simulink model "usv_6dof"  (R2023b)
settings: Solver=VariableStepAuto  StartTime=0.0  StopTime=200  RelTol=1e-3
libraries: slpidlib x1
settings Model: Creator=hw  LastModifiedBy=hw

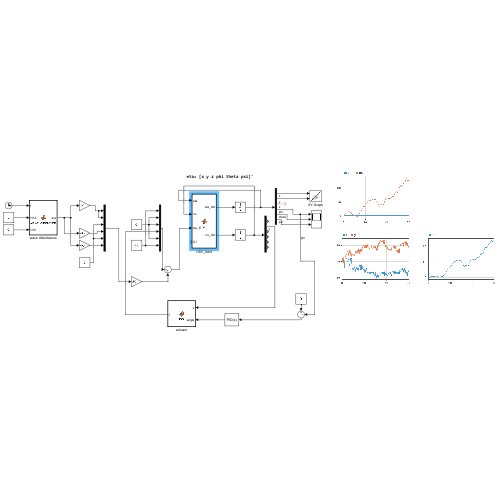
[thumbnail: Simulink's stored preview of the top-level diagram]
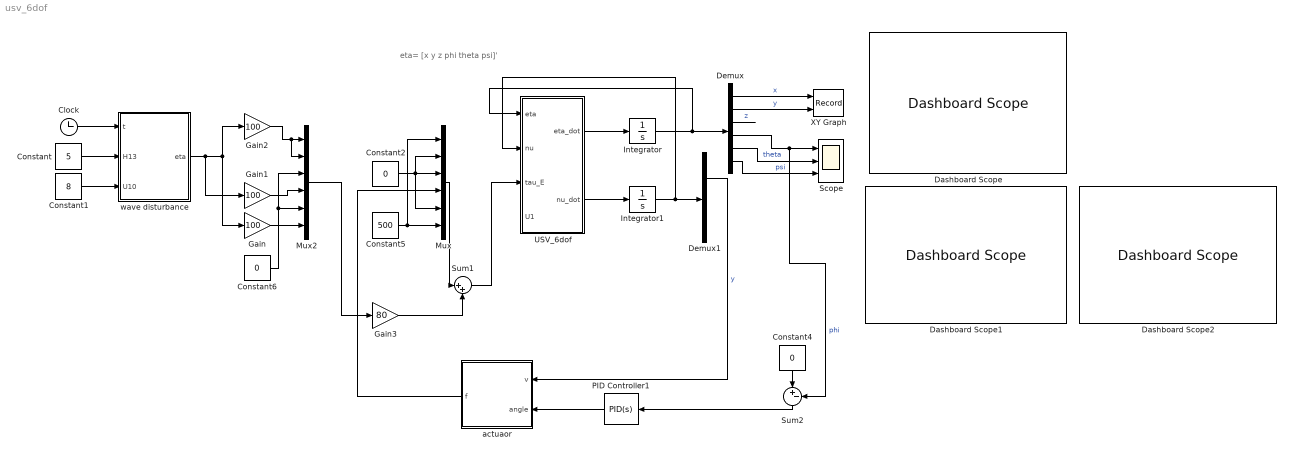
== system usv_6dof ==
  note: eta= [x y z phi theta psi]'
  Clock : Clock
  Constant : Constant  Value=5
  Constant1 : Constant  Value=8
  Constant2 : Constant  Value=0
  Constant4 : Constant  Value=0
  Constant5 : Constant  Value=500
  Constant6 : Constant  Value=0
  Dashboard Scope : DashboardScope
  Dashboard Scope1 : DashboardScope
  Dashboard Scope2 : DashboardScope
  Demux : Demux  Outputs=6
  Demux1 : Demux  Outputs=6
  Gain : Gain  Gain=100
  Gain1 : Gain  Gain=100
  Gain2 : Gain  Gain=100
  Gain3 : Gain  Gain=80
  Integrator : Integrator
  Integrator1 : Integrator
  Mux : Mux  Inputs=6
  Mux2 : Mux  Inputs=6
  PID Controller1 : slpidlib/PID Controller  Controller=PID  Form=Parallel  TimeDomain=Continuous-time  UseExternalTs=off  SampleTime=-1  IntegratorMethod=Forward Euler  FilterMethod=Forward Euler  ControllerParametersSource=internal  P=5  I=3  UseKiTs=off  D=2  N=100  UseFilter=on  TunerSelectOption=Transfer Function Based (PID Tuner App)  InitialConditionSource=internal  InitialConditionForIntegrator=0  InitialConditionForFilter=0  DifferentiatorICPrevScaledInput=0  ExternalReset=none  TrackingMode=off  Kt=1  LimitOutput=off  SatLimitsSource=internal  UpperSaturationLimit=inf  LowerSaturationLimit=-inf  LinearizeAsGain=on  AntiWindupMode=none  Kb=1  LimitIntegrator=off  UpperIntegratorSaturationLimit=inf  LowerIntegratorSaturationLimit=-inf  POutMin=[]  POutMax=[]  IOutMin=[]  IOutMax=[]  DOutMin=[]  DOutMax=[]  NOutMin=[]  NOutMax=[]  SumOutMin=[-15]  SumOutMax=[15]  SaturationOutMin=[]  SaturationOutMax=[]  PParamMin=[]  PParamMax=[]  IParamMin=[]  IParamMax=[]  DParamMin=[]  DParamMax=[]  NParamMin=[]  NParamMax=[]  KbParamMin=[]  KbParamMax=[]  KtParamMin=[]  KtParamMax=[]  KbOutMin=[]  KbOutMax=[]  KtOutMin=[]  KtOutMax=[]  IntegratorOutMin=[]  IntegratorOutMax=[]  FilterOutMin=[]  FilterOutMax=[]  SumI1OutMin=[]  SumI1OutMax=[]  SumI2OutMin=[]  SumI2OutMax=[]  SumI3OutMin=[]  SumI3OutMax=[]  SumI4OutMin=[]  SumI4OutMax=[]  SumDOutMin=[]  SumDOutMax=[]  DifferentiatorOutMin=[]  DifferentiatorOutMax=[]  FilterDiffOutCoefMin=[]  FilterDiffOutCoefMax=[]  ReciprocalOutMin=[]  ReciprocalOutMax=[]  SumDenOutMin=[]  SumDenOutMax=[]  SumNumOutMin=[]  SumNumOutMax=[]  DivideOutMin=[]  DivideOutMax=[]  UdiffTsProdOutMin=[]  UdiffTsProdOutMax=[]  NTsProdOutMin=[]  NTsProdOutMax=[]  UintegralTsProdOutMin=[]  UintegralTsProdOutMax=[]  UngainTsProdOutMin=[]  UngainTsProdOutMax=[]  ClampingZeroOutDataTypeStr=Inherit: Inherit via back propagation  ClampingZeroOutMin=[]  ClampingZeroOutMax=[]  FilterDenConstantOutDataTypeStr=Inherit: Inherit via back propagation  FilterDenConstantOutMin=[]  FilterDenConstantOutMax=[]  PCopyOutDataTypeStr=Inherit: Inherit via back propagation  PCopyOutMin=[]  PCopyOutMax=[]  NCopyOutDataTypeStr=Inherit: Inherit via back propagation  NCopyOutMin=[]  NCopyOutMax=[]  IntegratorContinuousStateAttributes=''  IntegratorStateMustResolveToSignalObject=off  IntegratorRTWStateStorageClass=Auto  FilterContinuousStateAttributes=''  FilterStateMustResolveToSignalObject=off  FilterRTWStateStorageClass=Auto  ParallelPVariant=InternalParameters  IdealPVariant=Disabled  IVariant=InternalParameters  DVariant=InternalParameters  IntegratorVariant=Continuous  SatVariant=Disabled  AWVariant=Passthrough  PCopyVariant=Disabled  TRVariant=Disabled  FdbkBlocksVariant=Forward  IdealPFdbkVariant=Disabled  SatFdbkVariant=Disabled  DerivativeFilterVariant=ContFilter  NVariant=InternalParameters  NCopyVariant=Disabled  FilterICVariant=InternalICsFilter  IntegratorICVariant=InternalICs  ExternalResetVariant=Disabled  TRSumVariant=Passthrough  SumFdbkVariant=Disabled  SumVariant=Sum_PID  TsampFilterVariant=InternalTs  TsampNgainVariant=Passthrough  TsampIntegralVariant=Disabled_SignalSpec  ExternalSaturationOutDataTypeStr=Inherit: Same as second input
  Scope : Scope  NumInputPorts=3
  Sum1 : Sum  Inputs=|++
  Sum2 : Sum  Inputs=|+-
  USV_6dof : MATLAB Function  TreatAsAtomicUnit=on
  XY Graph : Record  FileSettingsInternal="{\"entries\":[{\"content\":{\"excelSettings\":{\"content\":{},\"type\":\"Streamout.ExcelSettings\"}},\"type\":\"Streamout.FileSettingStorage\",\"uuid\":\"\"}],\"packageUris\":[\"http:\\/\\/schema.mathworks.com\\/mf0\\/streamout_blocks\\/R2020a\"],\"version\":\"1.0\"}"  Layout=[1 1]  SignalsInternal="{\"entries\":[{\"content\":{\"signals\":[{\"content\":{\"blockPath\":[],\"dimensions\":[1],\"domain\":\"\",\"lineColor\":\"#a2142f\",\"plots\":[1],\"port\":1,\"sid\":[\"\"],\"signalID\":11724,\"signalName\":\"x\"},\"type\":\"RecordBlkView.Signal\",\"uuid\":\"\"},{\"content\":{\"blockPath\":[],\"dimensions\":[1],\"domain\":\"\",\"lineColor\":\"#139fff\",\"plots\":[1],\"port\":2,\"sid\":[\"\"],\"signalID\":11728,\"signalName\":\"y\"},\"type\":\"RecordBlkView.Signal\",\"uuid\":\"\"}]},\"type\":\"RecordBlkView.InputSignals\",\"uuid\":\"\"}],\"packageUris\":[\"http:\\/\\/schema.mathworks.com\\/mf0\\/streamout_blocks\\/R2020a\"],\"version\":\"1.0\"}"  VisualizationBindings="{\"xyplotplugin\":{\"info\":[{\"series\":[{\"bindingParametersList\":[{\"parameter\":\"X-Axis\",\"signalID\":11724,\"signalName\":\"x\"},{\"parameter\":\"Y-Axis\",\"signalID\":11728,\"signalName\":\"y\"}],\"seriesID\":30360}],\"subplotID\":1}]}}"  CompatibilityTag=XY
  actuaor : MATLAB Function  TreatAsAtomicUnit=on
  wave disturbance : MATLAB Function  TreatAsAtomicUnit=on
  wires:
  wave disturbance/1(eta) -> Gain1/1, Gain2/1, Gain/1
  USV_6dof/2(nu_dot) -> Integrator1/1
  Constant/1 -> wave disturbance/2(H13)
  Integrator1/1 -> Demux1/1, USV_6dof/2(nu)
  Integrator/1 -> USV_6dof/1(eta), Demux/1
  Clock/1 -> wave disturbance/1(t)
  USV_6dof/1(eta_dot) -> Integrator/1
  Constant1/1 -> wave disturbance/3(U10)
  Demux/1 -> XY Graph/1  "x"
  Demux/2 -> XY Graph/2  "y"
  Demux/3 -> ?  "z"
  Demux/5 -> Scope/2  "theta"
  Demux/6 -> Scope/3  "psi"
  Constant2/1 -> Mux/5, Mux/2, Mux/3
  Constant5/1 -> Mux/6, Mux/1
  Mux/1 -> Sum1/1
  Gain2/1 -> Mux2/2, Mux2/1
  Gain/1 -> Mux2/6
  Mux2/1 -> Gain3/1
  Sum1/1 -> USV_6dof/3(tau_E)
  Gain1/1 -> Mux2/4
  Constant6/1 -> Mux2/5, Mux2/3
  Gain3/1 -> Sum1/2
  actuaor/1(f) -> Mux/4
  PID Controller1/1 -> actuaor/2(angle)
  Constant4/1 -> Sum2/1
  Demux/4 -> Sum2/2, Scope/1  "phi"
  Sum2/1 -> PID Controller1/1
  Demux1/2 -> actuaor/1(v)  "y"

== matlab function usv_6dof/actuaor ==
  data: v input; angle input size=1*1; f output size=1*1
function f  = top(v, angle)

f=1/2*v^2*1025*angle*10;
end

== matlab function usv_6dof/USV_6dof ==
  data: eta input size=6*1; eta_dot output size=6*1; nu input size=6*1; nu_dot output size=6*1; tau_E input size=6*1; U1 input
function [eta_dot,nu_dot]= fcn(eta,nu,tau_E,U1)
%%定义常量
    m=37;     %船体质量
    g = 9.81; % 重力加速度, m/s^2
    rho = 1025; % 海水密度, kg/m^3
    r_G=[0,0,0]'; %质心坐标
    r_f=[0 0 0]';  %浮心坐标
    I0=[0.11 0.11 0.11;0.22 0.22 0.22;0.33 0.33 0.33];  %转动惯量
    V=0.4562;  %排水体积
    W=m*g;
    B=W;
    % % B=rho*g*V;
%%定义位置与姿态等
    x=eta(1);
    y=eta(2);
    z=eta(3);
    phi=eta(4);
    theta=eta(5);
    psi=eta(6);

    u=nu(1);
    v=nu(2);
    w=nu(3);
    p=nu(4);
    q=nu(5);
    r=nu(6);
    
    x_g=r_G(1);
    y_g=r_G(2);
    z_g=r_G(3);

    x_f=r_f(1);
    y_f=r_f(2);
    z_f=r_f(3);

    % 转动惯量
    I_x = I0(1,1); % 绕x轴的转动惯量
    I_y = I0(2,2); % 绕y轴的转动惯量
    I_z = I0(3,3); % 绕z轴的转动惯量
    I_xy = -I0(1,2); % x-y平面的惯性积
    I_xz = -I0(1,3); % x-z平面的惯性积
    I_yz = -I0(2,3); % y-z平面的惯性积
%%定义转换矩阵
    J_eta = [cos(psi)*cos(theta), -sin(psi)*cos(phi) + cos(psi)*sin(theta)*sin(phi), sin(psi)*sin(phi) + cos(psi)*cos(phi)*sin(theta),0,0,0;
              sin(psi)*cos(theta), cos(psi)*cos(phi) + sin(psi)*sin(theta)*sin(phi), -cos(psi)*sin(phi) + sin(psi)*cos(phi)*sin(theta),0,0,0;
              -sin(theta), cos(theta)*sin(phi), cos(theta)*cos(phi),0,0,0;
              0,0,0,1,sin(phi)*tan(theta),cos(phi)*tan(theta);
              0,0,0,0,cos(phi),-sin(phi);
              0,0,0,0,sin(phi)/cos(theta),cos(phi)/cos(theta)]; 
  % 刚体质量矩阵
    M_RB = [
        m,   0,   0,   0,  m*z_g, -m*y_g;
        0,   m,   0,  -m*z_g, 0,  m*x_g;
        0,   0,   m,  m*y_g, -m*x_g, 0;
        0,  -m*z_g, m*y_g, I_x, -I_xy, -I_xz;
        m*z_g, 0,  -m*x_g, -I_xy, I_y, -I_yz;
        -m*y_g, m*x_g, 0, -I_xz, -I_yz, I_z];
  
   
        A11 =1000;  % 附加质量，沿x轴
        A22 = 1000;  % 附加质量，沿y轴
        A33 = 1000;  % 附加质量，沿z轴
        A44 = 1000;   % 附加转动惯量，绕x轴
        A55 =  1000;   % 附加转动惯量，绕y轴
        A66 =  1000;   % 附加转动惯量，绕z轴
        
        % 附加质量矩阵通常是对称的，非对角线上的值通常较小或为零
        M_A = diag([A11, A22, A33, A44, A55, A66]);
  % 根据提供的公式构造科里奥利和离心力矩阵
    C_RB = [
        0, 0, 0,  m*(y_g*q + z_g*r), -m*(x_g*q - w), -m*(x_g*r +v);
        0, 0, 0, -m*(y_g*p + w), m*(z_g*r + x_g*p),-m*(y_g*r - u);
        0, 0, 0, -m*(z_g*p - v), -m*(z_g*q + u), m*(x_g*p+y_g*q);
        -m*(y_g*q + z_g*r) , m*(y_g*p + w),m*(z_g*p - v) , 0 , -I_yz*q-I_xz*p+I_z*r, I_yz*r+I_xy*p-I_y*q ;
        m*(x_g*q - w) , -m*(z_g*r + x_g*p), m*(z_g*q + u),I_yz*q+I_xz*p-I_z*r,0, -I_xz*r-I_xy*q+I_x*p;
        m*(x_g*r +v), m*(y_g*r - u), -m*(x_g*p+y_g*q), -I_yz*r-I_xy*p+I_y*q ,I_xz*r+I_xy*q-I_x*p,0;
    ];    
    
    C_A =M_A;  % 附加科里奥利力和离心力矩阵
    % 船舶的阻尼系数，单位为 N·s/m 和 N·m·s/rad
    D_linear = [150, 0, 0, 0, 0, 0;  % 沿x方向的线性阻尼
                0, 150, 0, 0, 0, 0;  % 沿y方向的线性阻尼
                0, 0, 150, 0, 0, 0;  % 沿z方向的线性阻尼
                0, 0, 0, 10, 0, 0;   % 绕x轴的旋转线性阻尼
                0, 0, 0, 0,10, 0;   % 绕y轴的旋转线性阻尼
                0, 0, 0, 0, 0, 1000];  % 
    
    % 重力和浮力矢量
    g_eta = [
        (W - B) * sin(theta);
        -(W - B) * cos(theta) * sin(phi);
        -(W - B) * cos(theta) * cos(phi);
        -(y_g * W - y_f * B) * cos(theta) * cos(phi) + (z_g * W - z_f * B) * cos(theta) * sin(phi);
        (z_g * W - z_f * B) * sin(theta) + (x_g * W - x_f * B) * cos(theta) * cos(phi);
        -(x_g * W - x_f * B) * cos(theta) * sin(phi) - (y_g * W - y_f * B) * sin(theta)
    ];  
    M=M_RB+M_A;
    C_nu=C_RB+C_A;
    E= [1,1,1,1,1,1]';
%%动力学&运动学模型
    eta_dot=J_eta*nu;
    nu_dot = M \ (-C_nu * nu - D_linear * nu - g_eta + tau_E);
end

== matlab function usv_6dof/wave disturbance ==
  settings: updateMethod=DISCRETE
  data: t input; eta output; H13 input; U10 input
function eta = waveGeneration(t, H13, U10)
    % 此函数根据给定的有效波高和风速生成海浪信号
    % 常数定义
    g = 9.81; % 重力加速度, m/s^2
    alpha = 8.11e-3;
    beta = 3.11;
    
    % 风速对应的遭遇频率
    omega_e = 0.84 * (g / U10)^(1/3); % 峰值遭遇频率, rad/s

    % 频率范围和增量
    if H13 <= 2.5
        omegab=0.3;
        omegal =3.0;
        delta_omega = 0.1;
    elseif H13 <= 5.0
        omegab=0.25;
        omegal = 2.4;
        delta_omega = 0.08;
    else 
        omegab=0.1;
        omegal = 1.7;
        delta_omega = 0.06;
    end
    omega = omegab:delta_omega:omegal;

    % 能量密度谱 S(omega)
    S_omega = alpha * g^2 ./ omega.^5 .* exp(-beta ./ (H13^2 * omega.^4));
    
    % 振幅和相位
    a_omega = sqrt(2 * S_omega * delta_omega);
    phi = rand(1, length(omega)) * 2 * pi;

    % 海浪位移初始化
    eta = zeros(size(t));

    % 构建波形
    for i = 1:length(omega)
        eta = eta + a_omega(i) * cos(omega(i) * t + phi(i));
    end
end
